simulink model "simulation_pdy_v2"  (R2015a)
settings: Solver=ode45  StartTime=0.0  StopTime=8000.0  RelTol=1e-3
libraries: simulink x2
settings Model: Creator=MateusVendramini  LastModifiedBy=MateusVendramini
settings SolverCC: AlgebraicLoopSolver=LineSearch

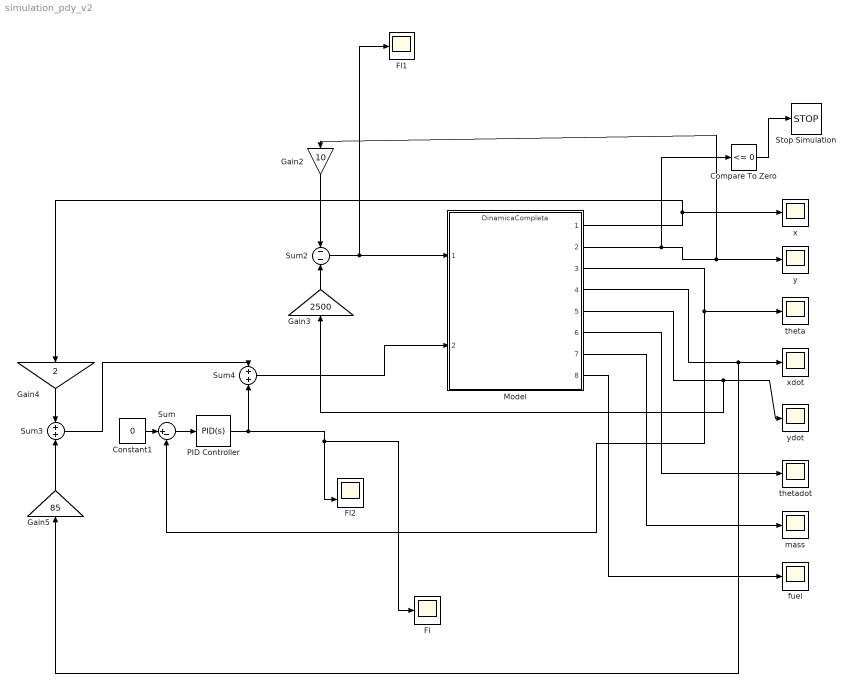
== system simulation_pdy_v2 ==
  Compare To Zero : simulink/Logic and Bit Operations/Compare To Zero  relop=<=  OutDataTypeStr=boolean
  Constant1 : Constant  Value=0
  Fl : Scope
      settings: SaveName=ScopeData8
  Fl1 : Scope
      settings: SaveName=ScopeData9
  Fl2 : Scope  NumInputPorts=2
      settings: YMin=-1000~-1000  YMax=1000~1000  SaveName=ScopeData10
  Gain2 : Gain  Gain=10
  Gain3 : Gain  Gain=2500
  Gain4 : Gain  Gain=2
  Gain5 : Gain  Gain=85
  Model : ModelReference  ModelNameDialog=DinamicaCompleta.slx  SimulationMode=Normal  ModelReferenceVersion=1.4  CopyOfModelName=DinamicaCompleta.slx  DefaultDataLogging=on
  PID Controller : simulink/Continuous/PID Controller  Controller=PID  TimeDomain=Continuous-time  SampleTime=-1  IntegratorMethod=Forward Euler  FilterMethod=Forward Euler  Form=Parallel  UseFilter=on  ControllerParametersSource=internal  P=2000  I=0  D=8500  N=100  InitialConditionSource=internal  InitialConditionForIntegrator=0  InitialConditionForFilter=0  ExternalReset=none  LimitOutput=off  UpperSaturationLimit=inf  LowerSaturationLimit=-inf  LinearizeAsGain=on  AntiWindupMode=none  Kb=1  TrackingMode=off  Kt=1  PParamMin=[]  PParamMax=[]  IParamMin=[]  IParamMax=[]  DParamMin=[]  DParamMax=[]  NParamMin=[]  NParamMax=[]  KbParamMin=[]  KbParamMax=[]  KtParamMin=[]  KtParamMax=[]  POutMin=[]  POutMax=[]  IOutMin=[]  IOutMax=[]  DOutMin=[]  DOutMax=[]  NOutMin=[]  NOutMax=[]  KbOutMin=[]  KbOutMax=[]  KtOutMin=[]  KtOutMax=[]  IntegratorOutMin=[]  IntegratorOutMax=[]  FilterOutMin=[]  FilterOutMax=[]  SumOutMin=[]  SumOutMax=[]  SumI1OutMin=[]  SumI1OutMax=[]  SumI2OutMin=[]  SumI2OutMax=[]  SumI3OutMin=[]  SumI3OutMax=[]  SumDOutMin=[]  SumDOutMax=[]  SaturationOutMin=[]  SaturationOutMax=[]  IntegratorContinuousStateAttributes=''  IntegratorStateMustResolveToSignalObject=off  IntegratorRTWStateStorageClass=Auto  FilterContinuousStateAttributes=''  FilterStateMustResolveToSignalObject=off  FilterRTWStateStorageClass=Auto  DifferentiatorICPrevScaledInput=0  DifferentiatorOutMin=[]  DifferentiatorOutMax=[]
  Stop Simulation : Stop
  Sum : Sum  Inputs=|+-
  Sum2 : Sum  Inputs=-|-
  Sum3 : Sum  Inputs=+|+
  Sum4 : Sum  Inputs=+|+
  fuel : Scope
      settings: TimeRange=16.32072553815624  YMin=700  YMax=891.0695187165775  SaveName=ScopeData7
  mass : Scope
      settings: SaveName=ScopeData6
  theta : Scope
      settings: SaveName=ScopeData2
  thetadot : Scope
      settings: SaveName=ScopeData5
  x : Scope
      settings: YMin=80  YMax=290
  xdot : Scope
      settings: SaveName=ScopeData3
  y : Scope
      settings: YMin=600000  YMax=2.4e+06
  ydot : Scope
      settings: SaveName=ScopeData4
  wires:
  Sum/1 -> PID Controller/1
  PID Controller/1 -> Fl2/2, Fl/1, Sum4/2
  Model/3 -> theta/1, Sum/2
  Model/1 -> Gain4/1, x/1
  Model/2 -> Compare To Zero/1, y/1, Gain2/1
  Model/4 -> xdot/1, Gain5/1
  Model/5 -> Gain3/1, ydot/1
  Model/6 -> thetadot/1
  Model/7 -> mass/1
  Model/8 -> fuel/1
  Gain2/1 -> Sum2/1
  Gain3/1 -> Sum2/2
  Sum2/1 -> Fl1/1, Model/1
  Compare To Zero/1 -> Stop Simulation/1
  Gain5/1 -> Sum3/2
  Gain4/1 -> Sum3/1
  Sum3/1 -> Sum4/1
  Constant1/1 -> Sum/1
  Sum4/1 -> Model/2
